simulink model "pt2_dc_machine"  (R2024b)
settings: Solver=ode15s  StartTime=0.0  StopTime=1  RelTol=1e-3
model workspace (MAT data in the model file):
  R = 10000
libraries: spsGroundLib x4, simulink x3, spsDCVoltageSourceLib x2, spsCurrentMeasurementLib x1, spsDCMachineLib x1, spsAsynchronousMachineSIUnitsLib x1, spsPowerLib x1, spsSeriesRLCBranchLib x1, spsThreePhaseSourceLib x1, spsVoltageMeasurementLib x1, sps_lib x1
settings Model: Creator=SIU856538288  LastModifiedBy=cloti
settings SolverCC: AlgebraicLoopSolver=TrustRegion
settings DebuggingCC: ArithmeticOperatorsInVariantConditions=warning
settings HardwareCC: ProdHWDeviceType=AMD->x86-64 (Windows64)
settings ModelReferenceCC: EnableRefExpFcnMdlSchedulingChecks=on
settings SFSimCC: CustomCodeUndefinedFunction=UseInterfaceOnly
settings RTWCC: GPUComputeCapability=3.5

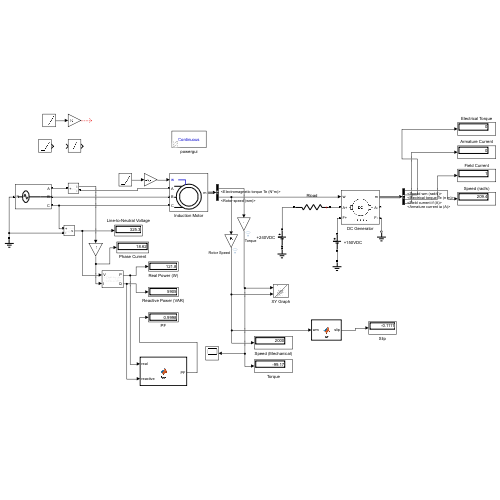
[thumbnail: Simulink's stored preview of the top-level diagram]
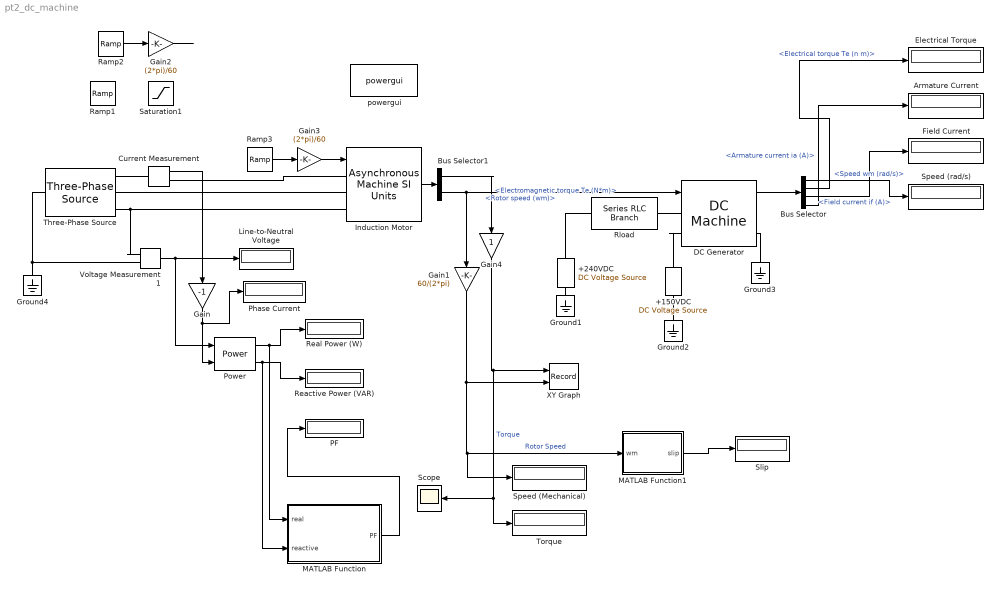
== system pt2_dc_machine ==
  +150VDC : spsDCVoltageSourceLib/DC Voltage Source  Amplitude=150  Measurements=Voltage
  +240VDC : spsDCVoltageSourceLib/DC Voltage Source  Amplitude=240  Measurements=Voltage
  Armature Current : Display
  Bus Selector : BusSelector  OutputSignals=Speed wm (rad/s),Electrical torque Te (n m),Field current if (A),Armature current ia (A)
  Bus Selector1 : BusSelector  OutputSignals=Mechanical.Electromagnetic torque Te (N*m),Mechanical.Rotor speed (wm)
  Current Measurement : spsCurrentMeasurementLib/Current Measurement  PhasorSimulation=off  OutputType=Complex  PSBequivalent=0
  DC Generator : spsDCMachineLib/DC Machine  PresetModel=02: 5HP 240V 1750RPM Field:150V  MechanicalLoad=Speed w  FieldType=Wound  ShowDetailedParameters=on  MeasurementBus=off  RLa=[0.78 0.016]  RLf=[150 112.5]  Laf=1.234  MachineConstant=Torque constant (N.m/A)  Ke=1.8  Kt=1.8  J=0.05  Bm=0.01  Tf=0  w0=1  Ifinit=1  TsPowergui=0  TsBlock=-1
  Electrical Torque : Display
  Field Current : Display
  Gain : Gain  Gain=-1
  Gain1 : Gain  Gain=60/(2*pi)
  Gain2 : Gain  Gain=(2*pi)/60
  Gain3 : Gain  Gain=(2*pi)/60
  Gain4 : Gain
  Ground{1..4} (4 alike) : spsGroundLib/Ground  LConnTagsString=a
  Induction Motor : spsAsynchronousMachineSIUnitsLib/Asynchronous Machine SI Units  RotorType=Squirrel-cage  PresetModel="01:  5 HP   460 V 60Hz 1750 RPM"  MechanicalLoad=Speed w  ShowDetailedParameters=on  ReferenceFrame=Rotor  Units=SI  MeasurementBus=off  NominalParameters=[3730 460 60]  VoltageRatio=1  Stator=[1.115 0.005974]  Rotor=[1.083 0.005974]  Cage1=[0.4155 0.002066]  Cage2=[0.4168 0.0003495]  Lm=0.2037  Mechanical=[0.02 0.005752 2]  PolePairs=2  InitialConditions=[0 0 0 0 0 0 0 0]  SimulateSaturation=off  Saturation=[14.03593122, 27.81365428, 53.79336849, 72.68890987, 97.98006896, 148.6815601, 215.7428561, 302.9841135, 428.7778367 ; 230, 322, 414, 460, 506, 552, 598, 644, 690]  LoadFlowParameters=1492000  TsPowergui=0  TsBlock=-1  IterativeModel=Trapezoidal non iterative  IterativeDiscreteModel=Trapezoidal non iterative  Pmec=1500
  Line-to-Neutral Voltage : Display
  MATLAB Function : MATLAB Function  TreatAsAtomicUnit=on
  MATLAB Function1 : MATLAB Function  TreatAsAtomicUnit=on
  PF : Display
  Phase Current : Display
  Power : spsPowerLib/Power  Freq=60  Vinit=[1, 0]  Iinit=[1, 0]  Ts=0
  Ramp1 : simulink/Sources/Ramp  slope=2000  start=0  InitialOutput=0  VectorParams1D=off
  Ramp2 : simulink/Sources/Ramp  slope=2000  start=0  InitialOutput=0  VectorParams1D=off
  Ramp3 : simulink/Sources/Ramp  slope=2000  start=0  InitialOutput=0  VectorParams1D=off
  Reactive Power (VAR) : Display
  Real Power (W) : Display
  Rload : spsSeriesRLCBranchLib/Series RLC Branch  LConnTagsString=__new0  RConnTagsString=__new0  BranchType=R  Resistance=100000  Inductance=1e-3  SetiL0=off  InitialCurrent=0  Capacitance=1e-6  Setx0=off  InitialVoltage=0  Measurements=None
  Saturation1 : Saturate  UpperLimit=1750
  Scope : Scope
  Slip : Display
  Speed (Mechanical) : Display
  Speed (rad/s) : Display
  Three-Phase Source : spsThreePhaseSourceLib/Three-Phase Source  InternalConnection=Yn  VoltagePhases=on  Voltage=265.58  PhaseAngle=0  Voltage_phases=[460 460 460]/sqrt(3)  PhaseAngles_phases=[0 -120 +120]  Frequency=60  NonIdealSource=on  SpecifyImpedance=off  Resistance=0  Inductance=0  ShortCircuitLevel=100e6  BaseVoltage=260  XRratio=7  BusType=swing  Pref=10e3  Qref=0  Prefabc=[10e3, 10e3, 10e3]  Qrefabc=[0, 0, 0]  Qmin=-inf  Qmax=inf
  Torque : Display
  Voltage Measurement1 : spsVoltageMeasurementLib/Voltage Measurement  PhasorSimulation=off  OutputType=Complex  PSBequivalent=0
  XY Graph : Record  FileSettingsInternal="{\"entries\":[{\"content\":{\"excelSettings\":{\"content\":{},\"type\":\"Streamout.ExcelSettings\"}},\"type\":\"Streamout.FileSettingStorage\",\"uuid\":\"\"}],\"packageUris\":[\"http:\\/\\/schema.mathworks.com\\/mf0\\/streamout_blocks\\/R2020a\"],\"version\":\"1.0\"}"  Layout=[1 1]  SignalsInternal="{\"entries\":[{\"content\":{\"signals\":[{\"content\":{\"blockPath\":[],\"dimensions\":[1],\"domain\":\"\",\"lineColor\":\"#a2142f\",\"plots\":[ 1 ],\"port\":1,\"sid\":[\"\"],\"signalID\":1,\"signalName\":\"Torque\"},\"type\":\"RecordBlkView.Signal\",\"uuid\":\"\"},{\"content\":{\"blockPath\":[],\"dimensions\":[1],\"domain\":\"\",\"lineColor\":\"#139fff\",\"plots\":[ 1 ],\"port\":2,\"sid\":[\"\"],\"signalID\":2,\"signalName\":\"Rotor Speed\"},\"type\":\"RecordBlkView.Signal\",\"uuid\":\"\"}]},\"type\":\"RecordBlkView.InputSignals\",\"uuid\":\"\"}],\"packageUris\":[\"http:\\/\\/schema.mathworks.com\\/mf0\\/streamout_blocks\\/R2020a\"],\"version\":\"1.0\"}"  VisualizationBindings="{\"xyplotplugin\":{\"info\":[{\"series\":[{\"bindingParametersList\":[{\"parameter\":\"X-Axis\",\"signalID\":2,\"signalName\":\"Rotor Speed\"},{\"parameter\":\"Y-Axis\",\"signalID\":1,\"signalName\":\"Torque\"},{\"parameter\":\"X-Axis\",\"signalID\":2,\"signalName\":\"Rotor Speed\"},{\"parameter\":\"Y-Axis\",\"signalID\":1,\"signalName\":\"Torque\"},{\"parameter\":\"X-Axis\",\"signalID\":2,\"signalName\":\"Rotor Speed\"},{\"parameter\":\"Y-Axis\",\"signalID\":1,\"signalName\":\"Torque\"}],\"seriesID\":0}],\"subplotID\":1}]}}"  CompatibilityTag=XY
  powergui : sps_lib/powergui  Priority=1  SimulationMode=Continuous  SampleTime=50e-6  frequency=60  Iterations=50  frequencyindice=60  Pbase=100e6  ErrMax=1e-4  UnitsV=kV  UnitsW=MW  buscounter=0  FunctionMessages=off  echomessages=off  EnableUseOfTLC=off  CurrentSourceSwitches=off  DisableSnubberDevices=off  DisableRonSwitches=off  DisableVfSwitches=off  DisplayEquations=off  AutomaticDiscreteSolvers=off  SolverType=Tustin/Backward Euler (TBE)  Interpol=off  ExternalGateDelay=off  methode=off  Ts=100  x0status=blocks  SPID=on  SwTol=0  HookPort=off  NonlinearTolerance=1e-4  nMaxIteration=100  ContinueOnMaxIteration=off  RestoreLinks=warning  ResistiveCurrentMeasurement=off  Frange=[0:2:500]  Ylog=off  Xlog=on  ShowGrid=off  save=off  variable=ZData  structure=0  ZoomFFT=off  StartTime=0.0  cycles=1  DisplayStyle=1  fundamental=60  FreqAxis=off  MaxFrequency=1000  frequencyindicesteady=1  RmsSteady=1  display=off
  wires:
  Induction Motor/1 -> Bus Selector1/1
  Current Measurement/1 -> Gain/1
  Power/2 -> MATLAB Function/2(reactive), Reactive Power (VAR)/1
  Power/1 -> MATLAB Function/1(real), Real Power (W)/1
  MATLAB Function/1(PF) -> PF/1
  Voltage Measurement1/1 -> Power/1, Line-to-Neutral Voltage/1
  Gain/1 -> Power/2, Phase Current/1
  MATLAB Function1/1(slip) -> Slip/1
  Bus Selector1/1 -> Gain4/1  "<Electromagnetic torque Te (N*m)>"
  DC Generator/1 -> Bus Selector/1
  Bus Selector1/2 -> DC Generator/1, Gain1/1  "<Rotor speed (wm)>"
  Bus Selector/2 -> Electrical Torque/1  "<Electrical torque Te (n m)>"
  Bus Selector/1 -> Speed (rad/s)/1  "<Speed wm (rad/s)>"
  Bus Selector/3 -> Field Current/1  "<Field current if (A)>"
  Bus Selector/4 -> Armature Current/1  "<Armature current ia (A)>"
  Gain1/1 -> XY Graph/2, Speed (Mechanical)/1, MATLAB Function1/1(wm)  "Rotor Speed"
  Gain4/1 -> XY Graph/1, Scope/1, Torque/1  "Torque"
  Ramp3/1 -> Gain3/1
  Gain3/1 -> Induction Motor/1
  Gain2/1 -> ?
  Ramp2/1 -> Gain2/1
  connections:
  Three-Phase Source/RConn2 -- Induction Motor/LConn2
  Three-Phase Source/RConn3 -- Voltage Measurement1/LConn1 -- Induction Motor/LConn3
  Voltage Measurement1/LConn2 -- Three-Phase Source/LConn1 -- Ground4/LConn1
  Three-Phase Source/RConn1 -- Current Measurement/LConn1
  Current Measurement/RConn1 -- Induction Motor/LConn1
  Ground3/LConn1 -- DC Generator/RConn2
  DC Generator/LConn1 -- Rload/LConn1
  Rload/RConn1 -- +240VDC/RConn1
  Ground2/LConn1 -- +150VDC/LConn1
  DC Generator/LConn2 -- +150VDC/RConn1
  Ground1/LConn1 -- +240VDC/LConn1

== matlab function pt2_dc_machine/MATLAB Function ==
  data: real input; PF output; reactive input
function PF = fcn(real, reactive)

PF = cos(atan(real/reactive));

== matlab function pt2_dc_machine/MATLAB Function1 ==
  data: wm input; slip output
function slip = fcn(wm)

ws = 1800;
slip = (ws-wm)/ws;
